simulink model "PMSM_comparison_with_matlab"  (R2023a)
settings: Solver=VariableStepAuto  StartTime=0.0  StopTime=10  MaxStep=1.0E-5  RelTol=1e-3  EnableMultiTasking=on
values from neighbouring files (symbols this model uses):
  F = 7.59e-5    (= 7.59e-05)    [initialize_motor.m]
  flux = 0.1    [initialize_motor.m]
  J = 0.00012    [initialize_motor.m]
  Ld = 0.004    [initialize_motor.m]
  Lq = 0.0035    [initialize_motor.m]
  P = 6    [initialize_motor.m]
  Rs = 2.2    [initialize_motor.m]
undefined symbols (not defined in the file or in its folder): induction_motor, sin_cos_calculator
libraries: spsACVoltageSourceLib x3, spsPermanentMagnetSynchronousMachineLib x1, spsGroundLib x1, spsThreePhaseSeriesRLCLoadLib x1, sps_lib x1
Description:
  | This model implements the model of permanent magnet synchronous motor
  | and compare it with the matlab model for verification of correctness.
  | 
  | Created by:
  | 
  | Syed Abdul Rahman Kashif
  | UET, Lahore
settings Model: Creator=kashif  LastModifiedBy=Derrick Baalaboore
settings SolverCC: AlgebraicLoopSolver=TrustRegion
settings DataIOCC: LimitDataPoints=on  SaveFormat=Array  SignalLoggingSaveFormat=ModelDataLogs  ReturnWorkspaceOutputs=off
settings OptimizationCC: ExpressionDepthLimit=2147483647  InitFltsAndDblsToZero=on  LifeSpan=inf
settings DebuggingCC: SaveWithParameterizedLinksMsg=none  UnderspecifiedInitializationDetection=Classic  MergeDetectMultiDrivingBlocksExec=none  SolverPrmCheckMsg=warning  MultiTaskCondExecSysMsg=none  FcnCallInpInsideContextMsg=warning  UnconnectedInputMsg=warning  UnconnectedOutputMsg=warning  UnconnectedLineMsg=warning  StateNameClashWarn=warning  SFUnexpectedBacktrackingDiag=warning  SFNoUnconditionalDefaultTransitionDiag=warning  SFExecutionAtInitializationDiag=none  ArithmeticOperatorsInVariantConditions=warning
settings HardwareCC: ProdBitPerPointer=32  ProdBitPerSizeT=32  ProdBitPerPtrDiffT=32  ProdLargestAtomicFloat=None  ProdIntDivRoundTo=Undefined  ProdEndianess=Unspecified  ProdWordSize=32  ProdHWDeviceType=32-bit Generic
settings ModelReferenceCC: PropagateSignalLabelsOutOfModel=off
settings SFSimCC: SimUseLocalCustomCode=off  CustomCodeUndefinedFunction=UseInterfaceOnly
settings RTWCC: RTWUseLocalCustomCode=off
settings CodeAppCC: StateflowObjectComments=on
settings GRTTargetCC: TargetLangStandard=C89/C90 (ANSI)  CombineOutputUpdateFcns=off  GRTInterface=on
settings ConfigComp: CovMetricSettings=dw  CovSaveCumulativeToWorkspaceVar=on  CovSaveSingleToWorkspaceVar=on  CovExternalEMLEnable=off

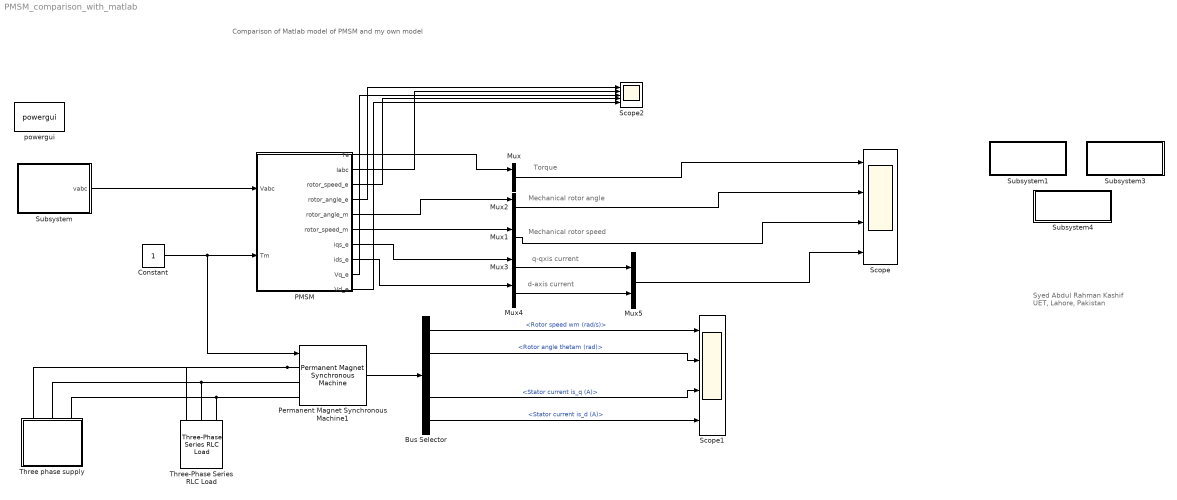
== system PMSM_comparison_with_matlab ==
  note: Torque
  note: Mechanical rotor angle
  note: Mechanical rotor speed
  note: q-qxis current
  note: d-axis current
  note: Comparison of Matlab model of PMSM and my own model
  note: Syed Abdul Rahman Kashif
      | UET, Lahore, Pakistan
  Bus Selector : BusSelector  OutputSignals=Rotor speed wm (rad/s),Rotor angle thetam (rad),Electromagnetic torque Te (N*m),Stator current is_q (A),Stator current is_d (A)
  Constant : Constant
  Mux{,1..5} (6 alike) : Mux  Inputs=2
  PMSM : Subsystem
  Permanent Magnet Synchronous Machine1 : spsPermanentMagnetSynchronousMachineLib/Permanent Magnet Synchronous Machine  NbPhases=3  FluxDistribution=Sinusoidal  RotorType=Salient-pole  MechanicalLoad=Torque Tm  PresetModel=No  ShowDetailedParameters=on  MeasurementBus=off  Resistance=1.6  Inductance=8.5e-3  dqInductances=[0.006365 0.006365]  La=0.000395  MachineConstant=Flux linkage established by magnets (V.s)  Flux=0.1852  VoltageCst=134.3663  TorqueCst=1.1112  Flat=120  Mechanical=[0.0001854 5.39e-5 4]  PolePairs=4  InitialConditions=[0,0, 0,0]  InitialConditions5ph=[0 0 0 0 0 0]  RefAngle=90 degrees behind phase A axis (modified Park)  IterativeDiscreteModel=Trapezoidal non iterative  TsBlock=-1  TsPowergui=0
  Scope : Scope  NumInputPorts=4
  Scope1 : Scope  NumInputPorts=4
  Scope2 : Scope  NumInputPorts=5
  Subsystem : Subsystem  mask{Vrms=220, f=50}
      mask prompts: f "frequency"
      mask Display: fprintf('Three phase \n Supply Vrms')
  Subsystem1 : Subsystem
      settings: OpenFcn=initialize_motor
      mask Display: fprintf('Initializing \n Data');
  Subsystem3 : Subsystem
      settings: OpenFcn=open('initialize_motor.m')
      mask Display: fprintf('Edit Data')
  Subsystem4 : Subsystem
      settings: OpenFcn=|
      | clear;
      | clc;
      | fprintf('All the Data has been cleared\n');
      mask Display: fprintf('Clear Data')
  Three phase supply : Subsystem  mask{Vrms=220, f=50}
      mask prompts: f "Frequency"
      mask Display: fprintf('Three phase \n Supply Vrms')
  Three-Phase Series RLC Load : spsThreePhaseSeriesRLCLoadLib/Three-Phase Series RLC Load  LConnTagsString=A|B|C  Configuration=Y (grounded)  NominalVoltage=220  Vabc=[1e3 1e3 1e3]  Vabcp=[1e3 1e3 1e3]  NominalFrequency=50  UnbalancedPower=off  ActivePower=100  InductivePower=0  CapacitivePower=0  Pabc=[10e3 9e3 11e3]  QLabc=[100 90 110]  QCabc=[100 90 110]  Pabcp=[10e3 9e3 11e3]  QLabcp=[100 90 110]  QCabcp=[100 90 110]  Measurements=None  LoadType=constant Z
  powergui : sps_lib/powergui  Priority=1  SimulationMode=Continuous  SampleTime=50e-6  frequency=60  Iterations=50  frequencyindice=50  Pbase=100e6  ErrMax=1e-4  UnitsV=kV  UnitsW=MW  buscounter=0  FunctionMessages=off  echomessages=off  EnableUseOfTLC=off  CurrentSourceSwitches=on  DisableSnubberDevices=off  DisableRonSwitches=off  DisableVfSwitches=off  DisplayEquations=off  AutomaticDiscreteSolvers=off  SolverType=Tustin/Backward Euler (TBE)  Interpol=off  ExternalGateDelay=off  methode=off  Ts=0  x0status=blocks  SPID=off  SwTol=0  HookPort=off  NonlinearTolerance=1e-4  nMaxIteration=100  ContinueOnMaxIteration=off  RestoreLinks=warning  ResistiveCurrentMeasurement=off  Frange=[0:2:500]  Ylog=off  Xlog=on  ShowGrid=off  save=off  variable=ZData  structure=0  ZoomFFT=on  StartTime=0.0  cycles=1  DisplayStyle=1  fundamental=60  FreqAxis=off  MaxFrequency=1000  frequencyindicesteady=1  RmsSteady=1  display=off
  wires:
  Subsystem/1(vabc) -> PMSM/1(Vabc)
  Permanent Magnet Synchronous Machine1/1 -> Bus Selector/1
  Mux/1 -> Scope/1
  Bus Selector/1 -> Scope1/1  "<Rotor speed wm (rad/s)>"
  Bus Selector/2 -> Scope1/2  "<Rotor angle thetam (rad)>"
  PMSM/1(Te) -> Mux/1
  Bus Selector/4 -> Scope1/3  "<Stator current is_q (A)>"
  Bus Selector/5 -> Scope1/4  "<Stator current is_d (A)>"
  PMSM/6(rotor_speed_m) -> Mux1/1
  PMSM/7(iqs_e) -> Mux3/1
  PMSM/5(rotor_angle_m) -> Mux2/1
  Mux2/1 -> Scope/2
  Mux1/1 -> Scope/3
  PMSM/8(ids_e) -> Mux4/1
  Mux3/1 -> Mux5/1
  Mux4/1 -> Mux5/2
  Mux5/1 -> Scope/4
  PMSM/2(Iabc) -> Scope2/2
  PMSM/3(rotor_speed_e) -> Scope2/4
  PMSM/4(rotor_angle_e) -> Scope2/1
  PMSM/9(Vq_e) -> Scope2/3
  PMSM/10(Vd_e) -> Scope2/5
  Constant/1 -> Permanent Magnet Synchronous Machine1/1, PMSM/2(Tm)
  connections:
  Permanent Magnet Synchronous Machine1/LConn1 -- Three phase supply/RConn1 -- Three-Phase Series RLC Load/LConn1
  Three phase supply/RConn2 -- Permanent Magnet Synchronous Machine1/LConn2 -- Three-Phase Series RLC Load/LConn2
  Three phase supply/RConn3 -- Permanent Magnet Synchronous Machine1/LConn3 -- Three-Phase Series RLC Load/LConn3

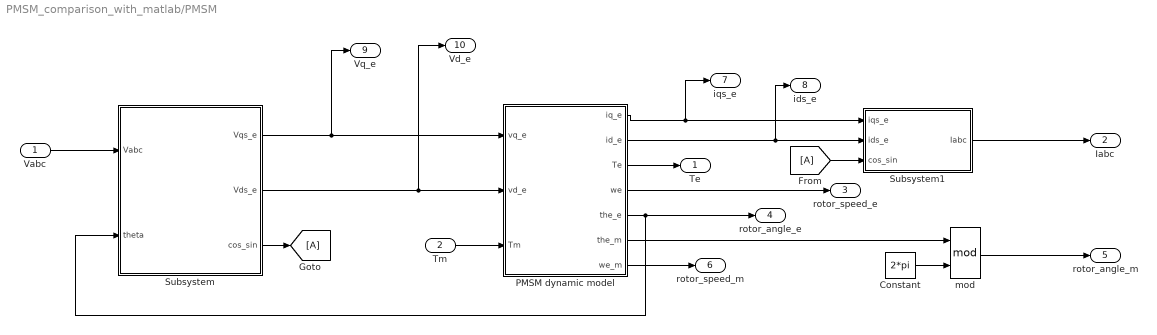
== system PMSM_comparison_with_matlab/PMSM ==
  Vabc : Inport
  Tm : Inport  Port=2
  Constant : Constant  Value=2*pi
  From : From
  Goto : Goto
  PMSM dynamic model : Subsystem
  Subsystem : Subsystem
  Subsystem1 : Subsystem
  mod : Math  Operator=mod  SignedPower=on
  Te : Outport
  Iabc : Outport  Port=2
  rotor_speed_e : Outport  Port=3
  rotor_angle_e : Outport  Port=4
  rotor_angle_m : Outport  Port=5
  rotor_speed_m : Outport  Port=6
  iqs_e : Outport  Port=7
  ids_e : Outport  Port=8
  Vq_e : Outport  Port=9
  Vd_e : Outport  Port=10
  wires:
  PMSM dynamic model/1(iq_e) -> iqs_e/1, Subsystem1/1(iqs_e)
  PMSM dynamic model/2(id_e) -> Subsystem1/2(ids_e), ids_e/1
  PMSM dynamic model/5(the_e) -> rotor_angle_e/1, Subsystem/2(theta)
  Subsystem/1(Vqs_e) -> Vq_e/1, PMSM dynamic model/1(vq_e)
  Subsystem/2(Vds_e) -> Vd_e/1, PMSM dynamic model/2(vd_e)
  PMSM dynamic model/4(we) -> rotor_speed_e/1
  PMSM dynamic model/3(Te) -> Te/1
  Vabc/1 -> Subsystem/1(Vabc)
  Tm/1 -> PMSM dynamic model/3(Tm)
  Subsystem1/1(Iabc) -> Iabc/1
  PMSM dynamic model/7(we_m) -> rotor_speed_m/1
  PMSM dynamic model/6(the_m) -> mod/1
  Constant/1 -> mod/2
  mod/1 -> rotor_angle_m/1
  Subsystem/3(cos_sin) -> Goto/1
  From/1 -> Subsystem1/3(cos_sin)

== system PMSM_comparison_with_matlab/Subsystem ==
  Mux : Mux  Inputs=3
  phase a : Sin  Amplitude=Vrms*sqrt(2)  Frequency=f*2*pi  SampleTime=0
  phase b : Sin  Amplitude=Vrms*sqrt(2)  Frequency=f*2*pi  Phase=240*pi/180  SampleTime=0
  phase c : Sin  Amplitude=Vrms*sqrt(2)  Frequency=f*2*pi  Phase=120*pi/180  SampleTime=0
  vabc : Outport
  wires:
  phase a/1 -> Mux/1
  phase b/1 -> Mux/2
  phase c/1 -> Mux/3
  Mux/1 -> vabc/1

== system PMSM_comparison_with_matlab/Subsystem1 ==

== system PMSM_comparison_with_matlab/Subsystem3 ==

== system PMSM_comparison_with_matlab/Subsystem4 ==

== system PMSM_comparison_with_matlab/Three phase supply ==
  Ground : spsGroundLib/Ground  LConnTagsString=a
  Va : spsACVoltageSourceLib/AC Voltage Source  Amplitude=Vrms*sqrt(2)  Phase=0  Frequency=f  SampleTime=0  Measurements=None  BusType=swing  Pref=10e3  Qref=0  Qmin=-inf  Qmax=+inf
  Vb : spsACVoltageSourceLib/AC Voltage Source  Amplitude=Vrms*sqrt(2)  Phase=240  Frequency=f  SampleTime=0  Measurements=None  BusType=swing  Pref=10e3  Qref=0  Qmin=-inf  Qmax=+inf
  Vc : spsACVoltageSourceLib/AC Voltage Source  Amplitude=Vrms*sqrt(2)  Phase=120  Frequency=f  SampleTime=0  Measurements=None  BusType=swing  Pref=10e3  Qref=0  Qmin=-inf  Qmax=+inf
  a : PMIOPort  Side=Right
  b : PMIOPort  Port=2  Side=Right
  c : PMIOPort  Port=3  Side=Right
  connections:
  Vb/LConn1 -- Va/LConn1 -- Ground/LConn1 -- Vc/LConn1
  a/RConn1 -- Va/RConn1
  b/RConn1 -- Vb/RConn1
  c/RConn1 -- Vc/RConn1

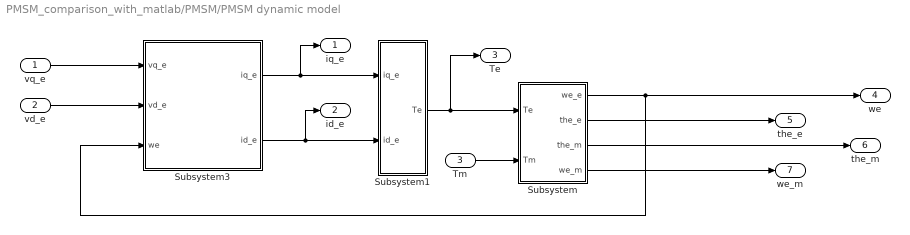
== system PMSM_comparison_with_matlab/PMSM/PMSM dynamic model ==
  vq_e : Inport
  vd_e : Inport  Port=2
  Tm : Inport  Port=3
  Subsystem : Subsystem
  Subsystem1 : Subsystem
  Subsystem3 : Subsystem
  iq_e : Outport
  id_e : Outport  Port=2
  Te : Outport  Port=3
  we : Outport  Port=4
  the_e : Outport  Port=5
  the_m : Outport  Port=6
  we_m : Outport  Port=7
  wires:
  Subsystem1/1(Te) -> Subsystem/1(Te), Te/1
  Subsystem3/1(iq_e) -> Subsystem1/1(iq_e), iq_e/1
  Subsystem3/2(id_e) -> Subsystem1/2(id_e), id_e/1
  Tm/1 -> Subsystem/2(Tm)
  vq_e/1 -> Subsystem3/1(vq_e)
  vd_e/1 -> Subsystem3/2(vd_e)
  Subsystem/2(the_e) -> the_e/1
  Subsystem/1(we_e) -> we/1, Subsystem3/3(we)
  Subsystem/3(the_m) -> the_m/1
  Subsystem/4(we_m) -> we_m/1

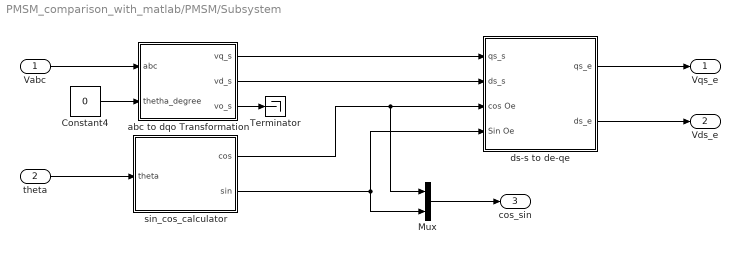
== system PMSM_comparison_with_matlab/PMSM/Subsystem ==
  Vabc : Inport
  theta : Inport  Port=2
  Constant4 : Constant  Value=0
  Mux : Mux  Inputs=2
  Terminator : Terminator
  abc to dqo Transformation : Subsystem  AncestorBlock=induction_motor/abc to dqo Transformation
      settings: LibrarySourceBlock=induction_motor/abc to dqo Transformation
  ds-s to de-qe : Subsystem  AncestorBlock=induction_motor/ds-s to de-qe
      settings: LibrarySourceBlock=induction_motor/ds-s to de-qe
  sin_cos_calculator : Subsystem  AncestorBlock=induction_motor/sin_cos_calculator
      settings: LibrarySourceBlock=induction_motor/sin_cos_calculator
  Vqs_e : Outport
  Vds_e : Outport  Port=2
  cos_sin : Outport  Port=3
  wires:
  abc to dqo Transformation/1(vq_s) -> ds-s to de-qe/1(qs_s)
  abc to dqo Transformation/2(vd_s) -> ds-s to de-qe/2(ds_s)
  Vabc/1 -> abc to dqo Transformation/1(abc)
  Constant4/1 -> abc to dqo Transformation/2(thetha_degree)
  ds-s to de-qe/1(qs_e) -> Vqs_e/1
  abc to dqo Transformation/3(vo_s) -> Terminator/1
  ds-s to de-qe/2(ds_e) -> Vds_e/1
  theta/1 -> sin_cos_calculator/1(theta)
  sin_cos_calculator/1(cos) -> ds-s to de-qe/3(cos Oe), Mux/1
  sin_cos_calculator/2(sin) -> ds-s to de-qe/4(Sin Oe), Mux/2
  Mux/1 -> cos_sin/1

== system PMSM_comparison_with_matlab/PMSM/Subsystem1 ==
  iqs_e : Inport
  ids_e : Inport  Port=2
  cos_sin : Inport  Port=3
  Constant2 : Constant  Value=0
  Demux : Demux  Outputs=2
  Subsystem : Subsystem
  de-qe to ds-qs : Subsystem  AncestorBlock=induction_motor/de-qe to ds-qs
      settings: LibrarySourceBlock=induction_motor/de-qe to ds-qs
  Iabc : Outport
  wires:
  de-qe to ds-qs/1(qs_s) -> Subsystem/1(q_s)
  de-qe to ds-qs/2(ds_s) -> Subsystem/2(d_s)
  Constant2/1 -> Subsystem/4(thetha_degree)
  Subsystem/1(abc) -> Iabc/1
  iqs_e/1 -> de-qe to ds-qs/1(qs_e)
  ids_e/1 -> de-qe to ds-qs/2(ds_e)
  Demux/1 -> de-qe to ds-qs/3(cos Oe)
  ? -> Subsystem/3(o_s)
  Demux/2 -> de-qe to ds-qs/4(Sin Oe)
  cos_sin/1 -> Demux/1

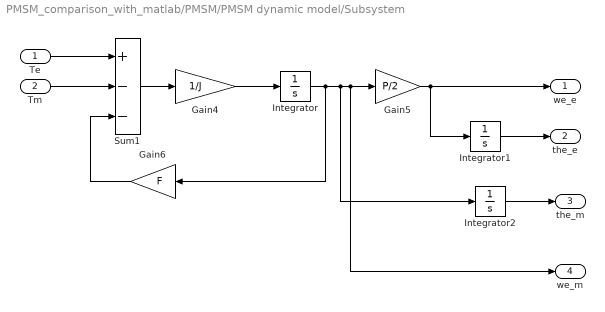
== system PMSM_comparison_with_matlab/PMSM/PMSM dynamic model/Subsystem ==
  Te : Inport
  Tm : Inport  Port=2
  Gain4 : Gain  Gain=1/J  SaturateOnIntegerOverflow=on  OutDataTypeStr=Inherit: Same as input  ParamDataTypeStr=Inherit: Same as input
  Gain5 : Gain  Gain=P/2  SaturateOnIntegerOverflow=on  OutDataTypeStr=Inherit: Same as input  ParamDataTypeStr=Inherit: Same as input
  Gain6 : Gain  Gain=F  SaturateOnIntegerOverflow=on  OutDataTypeStr=Inherit: Same as input  ParamDataTypeStr=Inherit: Same as input
  Integrator : Integrator
  Integrator1 : Integrator
  Integrator2 : Integrator
  Sum1 : Sum  Inputs=+--  InputSameDT=on  SaturateOnIntegerOverflow=on  OutDataTypeStr=Inherit: Same as first input
  we_e : Outport
  the_e : Outport  Port=2
  the_m : Outport  Port=3
  we_m : Outport  Port=4
  wires:
  Te/1 -> Sum1/1
  Tm/1 -> Sum1/2
  Sum1/1 -> Gain4/1
  Gain4/1 -> Integrator/1
  Integrator/1 -> Gain6/1, Integrator2/1, Gain5/1, we_m/1
  Gain6/1 -> Sum1/3
  Gain5/1 -> Integrator1/1, we_e/1
  Integrator1/1 -> the_e/1
  Integrator2/1 -> the_m/1

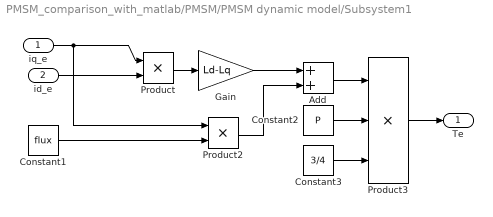
== system PMSM_comparison_with_matlab/PMSM/PMSM dynamic model/Subsystem1 ==
  iq_e : Inport
  id_e : Inport  Port=2
  Add : Sum
  Constant1 : Constant  Value=flux
  Constant2 : Constant  Value=P
  Constant3 : Constant  Value=3/4
  Gain : Gain  Gain=Ld-Lq
  Product : Product  RndMeth=Zero
  Product2 : Product  RndMeth=Zero
  Product3 : Product  Inputs=3  RndMeth=Zero
  Te : Outport
  wires:
  iq_e/1 -> Product/1, Product2/1
  id_e/1 -> Product/2
  Product/1 -> Gain/1
  Constant1/1 -> Product2/2
  Gain/1 -> Add/1
  Product2/1 -> Add/2
  Add/1 -> Product3/1
  Constant2/1 -> Product3/2
  Constant3/1 -> Product3/3
  Product3/1 -> Te/1

== system PMSM_comparison_with_matlab/PMSM/PMSM dynamic model/Subsystem3 ==
  vq_e : Inport
  vd_e : Inport  Port=2
  we : Inport  Port=3
  Subsystem1 : Subsystem
  Subsystem2 : Subsystem
  iq_e : Outport
  id_e : Outport  Port=2
  wires:
  vq_e/1 -> Subsystem1/3(vq)
  vd_e/1 -> Subsystem2/3(vd)
  we/1 -> Subsystem1/2(we), Subsystem2/2(we)
  Subsystem1/1(iq) -> Subsystem2/1(iq), iq_e/1
  Subsystem2/1(id) -> Subsystem1/1(id), id_e/1

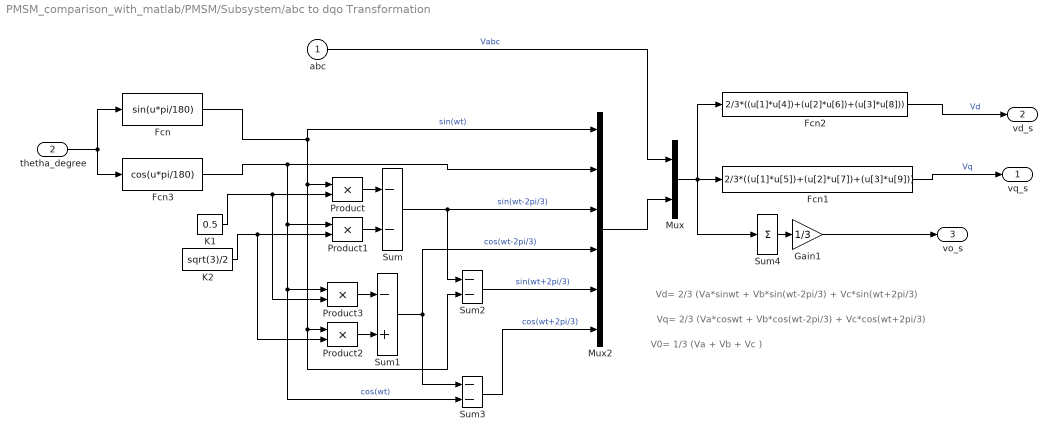
== system PMSM_comparison_with_matlab/PMSM/Subsystem/abc to dqo Transformation ==
  note: Vq= 2/3 (Va*coswt + Vb*cos(wt-2pi/3) + Vc*cos(wt+2pi/3)
  note: Vd= 2/3 (Va*sinwt + Vb*sin(wt-2pi/3) + Vc*sin(wt+2pi/3)
  note: V0= 1/3 (Va + Vb + Vc )
  abc : Inport  PortDimensions=3
  thetha_degree : Inport  Port=2
  Fcn : Fcn  Expr=sin(u*pi/180)
  Fcn1 : Fcn  Expr=2/3*((u[1]*u[5])+(u[2]*u[7])+(u[3]*u[9]))
  Fcn2 : Fcn  Expr=2/3*((u[1]*u[4])+(u[2]*u[6])+(u[3]*u[8]))
  Fcn3 : Fcn  Expr=cos(u*pi/180)
  Gain1 : Gain  Gain=1/3  SaturateOnIntegerOverflow=on  OutDataTypeStr=Inherit: Same as input  ParamDataTypeStr=Inherit: Same as input
  K1 : Constant  Value=0.5
  K2 : Constant  Value=sqrt(3)/2
  Mux : Mux  Inputs=2
  Mux2 : Mux  Inputs=6
  Product{,1..3} (4 alike) : Product  InputSameDT=on  SaturateOnIntegerOverflow=on  OutDataTypeStr=Inherit: Same as first input
  Sum : Sum  Inputs=--  InputSameDT=on  SaturateOnIntegerOverflow=on  OutDataTypeStr=Inherit: Same as first input
  Sum1 : Sum  Inputs=-+  InputSameDT=on  SaturateOnIntegerOverflow=on  OutDataTypeStr=Inherit: Same as first input
  Sum2 : Sum  Inputs=--  InputSameDT=on  SaturateOnIntegerOverflow=on  OutDataTypeStr=Inherit: Same as first input
  Sum3 : Sum  Inputs=--  InputSameDT=on  SaturateOnIntegerOverflow=on  OutDataTypeStr=Inherit: Same as first input
  Sum4 : Sum  Inputs=1  InputSameDT=on  SaturateOnIntegerOverflow=on  OutDataTypeStr=Inherit: Same as first input
  vq_s : Outport
  vd_s : Outport  Port=2
  vo_s : Outport  Port=3
  wires:
  Fcn2/1 -> vd_s/1  "Vd"
  Fcn1/1 -> vq_s/1  "Vq"
  abc/1 -> Mux/1  "Vabc"
  Mux2/1 -> Mux/2
  Fcn3/1 -> Sum3/2, Product3/1, Product1/1, Mux2/2  "cos(wt)"
  Fcn/1 -> Product/1, Product2/1, Sum2/2, Mux2/1  "sin(wt)"
  Product/1 -> Sum/1
  Product1/1 -> Sum/2
  Product3/1 -> Sum1/1
  Product2/1 -> Sum1/2
  Sum3/1 -> Mux2/6  "cos(wt+2pi/3)"
  Sum2/1 -> Mux2/5  "sin(wt+2pi/3)"
  K1/1 -> Product/2, Product3/2
  K2/1 -> Product1/2, Product2/2
  Sum/1 -> Mux2/3, Sum2/1  "sin(wt-2pi/3)"
  Sum1/1 -> Mux2/4, Sum3/1  "cos(wt-2pi/3)"
  Mux/1 -> Fcn2/1, Fcn1/1, Sum4/1
  Sum4/1 -> Gain1/1
  Gain1/1 -> vo_s/1
  thetha_degree/1 -> Fcn3/1, Fcn/1

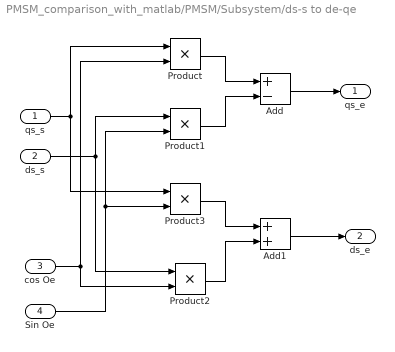
== system PMSM_comparison_with_matlab/PMSM/Subsystem/ds-s to de-qe ==
  qs_s : Inport
  ds_s : Inport  Port=2
  cos Oe : Inport  Port=3
  Sin Oe : Inport  Port=4
  Add : Sum  Inputs=+-
  Add1 : Sum
  Product{,1..3} (4 alike) : Product  RndMeth=Zero
  qs_e : Outport
  ds_e : Outport  Port=2
  wires:
  Product/1 -> Add/1
  Product1/1 -> Add/2
  Product2/1 -> Add1/2
  Product3/1 -> Add1/1
  Add1/1 -> ds_e/1
  Add/1 -> qs_e/1
  Sin Oe/1 -> Product1/2, Product3/2
  ds_s/1 -> Product1/1, Product2/1
  cos Oe/1 -> Product/2, Product2/2
  qs_s/1 -> Product/1, Product3/1

== system PMSM_comparison_with_matlab/PMSM/Subsystem/sin_cos_calculator ==
  theta : Inport
  Fcn : Fcn  Expr=sin(u)
  Fcn1 : Fcn  Expr=cos(u)
  cos : Outport
  sin : Outport  Port=2
  wires:
  Fcn1/1 -> cos/1
  Fcn/1 -> sin/1
  theta/1 -> Fcn/1, Fcn1/1

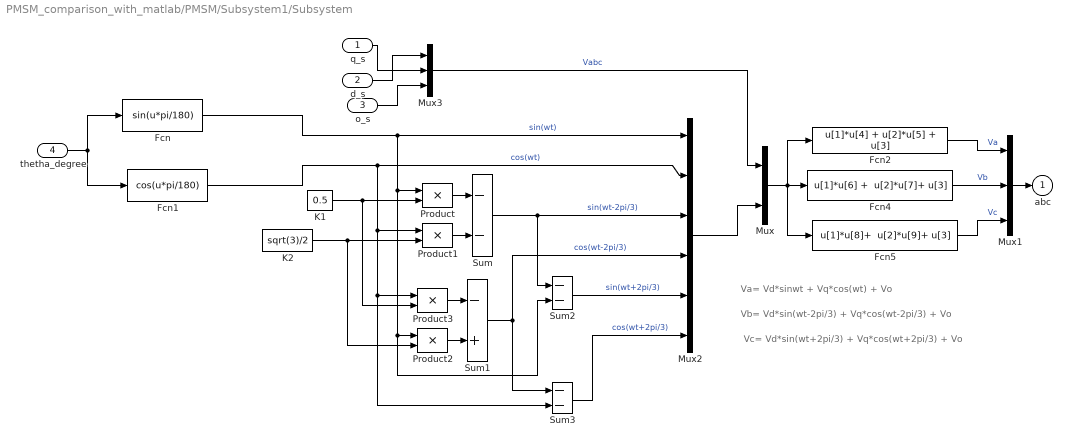
== system PMSM_comparison_with_matlab/PMSM/Subsystem1/Subsystem ==
  note: Va= Vd*sinwt + Vq*cos(wt) + Vo
  note: Vb= Vd*sin(wt-2pi/3) + Vq*cos(wt-2pi/3) + Vo
  note: Vc= Vd*sin(wt+2pi/3) + Vq*cos(wt+2pi/3) + Vo
  q_s : Inport
  d_s : Inport  Port=2
  o_s : Inport  Port=3
  thetha_degree : Inport  Port=4
  Fcn : Fcn  Expr=sin(u*pi/180)
  Fcn1 : Fcn  Expr=cos(u*pi/180)
  Fcn2 : Fcn  Expr="u[1]*u[4] +  u[2]*u[5] + u[3]"
  Fcn4 : Fcn  Expr="u[1]*u[6] +  u[2]*u[7]+ u[3]"
  Fcn5 : Fcn  Expr="u[1]*u[8]+  u[2]*u[9]+ u[3]"
  K1 : Constant  Value=0.5
  K2 : Constant  Value=sqrt(3)/2
  Mux : Mux  Inputs=2
  Mux1 : Mux  Inputs=3
  Mux2 : Mux  Inputs=6
  Mux3 : Mux  Inputs=3
  Product{,1..3} (4 alike) : Product  InputSameDT=on  SaturateOnIntegerOverflow=on  OutDataTypeStr=Inherit: Same as first input
  Sum : Sum  Inputs=--  InputSameDT=on  SaturateOnIntegerOverflow=on  OutDataTypeStr=Inherit: Same as first input
  Sum1 : Sum  Inputs=-+  InputSameDT=on  SaturateOnIntegerOverflow=on  OutDataTypeStr=Inherit: Same as first input
  Sum2 : Sum  Inputs=--  InputSameDT=on  SaturateOnIntegerOverflow=on  OutDataTypeStr=Inherit: Same as first input
  Sum3 : Sum  Inputs=--  InputSameDT=on  SaturateOnIntegerOverflow=on  OutDataTypeStr=Inherit: Same as first input
  abc : Outport  InitialOutput=0
  wires:
  o_s/1 -> Mux3/3
  q_s/1 -> Mux3/2
  d_s/1 -> Mux3/1
  Fcn5/1 -> Mux1/3  "Vc"
  Fcn2/1 -> Mux1/1  "Va"
  Mux1/1 -> abc/1
  Mux/1 -> Fcn4/1, Fcn2/1, Fcn5/1
  Sum1/1 -> Sum3/1, Mux2/4  "cos(wt-2pi/3)"
  Sum/1 -> Sum2/1, Mux2/3  "sin(wt-2pi/3)"
  K2/1 -> Product2/2, Product1/2
  K1/1 -> Product3/2, Product/2
  Sum2/1 -> Mux2/5  "sin(wt+2pi/3)"
  Sum3/1 -> Mux2/6  "cos(wt+2pi/3)"
  Product2/1 -> Sum1/2
  Product3/1 -> Sum1/1
  Product1/1 -> Sum/2
  Product/1 -> Sum/1
  Mux2/1 -> Mux/2
  Mux3/1 -> Mux/1  "Vabc"
  Fcn4/1 -> Mux1/2  "Vb"
  Fcn1/1 -> Mux2/2, Product1/1, Product3/1, Sum3/2  "cos(wt)"
  thetha_degree/1 -> Fcn/1, Fcn1/1
  Fcn/1 -> Mux2/1, Product/1, Sum2/2, Product2/1  "sin(wt)"

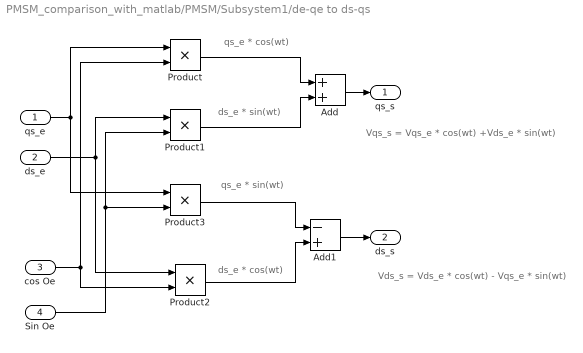
== system PMSM_comparison_with_matlab/PMSM/Subsystem1/de-qe to ds-qs ==
  note: Vds_s = Vds_e * cos(wt) - Vqs_e * sin(wt)
  note: Vqs_s = Vqs_e * cos(wt) +Vds_e * sin(wt)
  note: ds_e * cos(wt)
  note: qs_e * sin(wt)
  note: ds_e * sin(wt)
  note: qs_e * cos(wt)
  qs_e : Inport
  ds_e : Inport  Port=2
  cos Oe : Inport  Port=3
  Sin Oe : Inport  Port=4
  Add : Sum
  Add1 : Sum  Inputs=-+
  Product{,1..3} (4 alike) : Product  RndMeth=Zero
  qs_s : Outport
  ds_s : Outport  Port=2
  wires:
  Product/1 -> Add/1
  Product1/1 -> Add/2
  Product2/1 -> Add1/2
  Product3/1 -> Add1/1
  Add1/1 -> ds_s/1
  Add/1 -> qs_s/1
  Sin Oe/1 -> Product1/2, Product3/2
  ds_e/1 -> Product1/1, Product2/1
  cos Oe/1 -> Product/2, Product2/2
  qs_e/1 -> Product/1, Product3/1

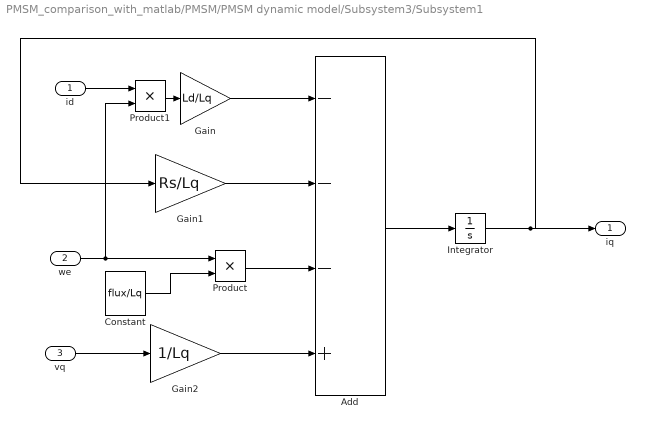
== system PMSM_comparison_with_matlab/PMSM/PMSM dynamic model/Subsystem3/Subsystem1 ==
  id : Inport
  we : Inport  Port=2
  vq : Inport  Port=3
  Add : Sum  Inputs=---+
  Constant : Constant  Value=flux/Lq
  Gain : Gain  Gain=Ld/Lq
  Gain1 : Gain  Gain=Rs/Lq
  Gain2 : Gain  Gain=1/Lq
  Integrator : Integrator
  Product : Product  RndMeth=Zero
  Product1 : Product  RndMeth=Zero
  iq : Outport
  wires:
  vq/1 -> Gain2/1
  Gain/1 -> Add/1
  Gain1/1 -> Add/2
  Gain2/1 -> Add/4
  Add/1 -> Integrator/1
  Integrator/1 -> Gain1/1, iq/1
  Product/1 -> Add/3
  we/1 -> Product/1, Product1/2
  Constant/1 -> Product/2
  Product1/1 -> Gain/1
  id/1 -> Product1/1

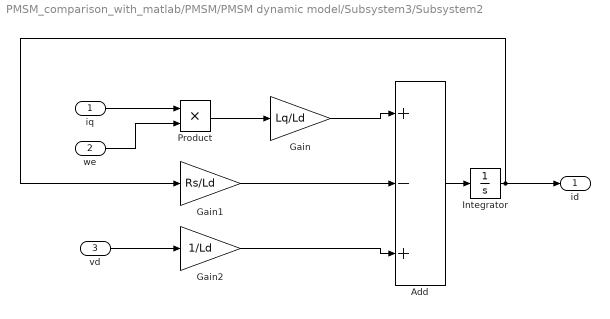
== system PMSM_comparison_with_matlab/PMSM/PMSM dynamic model/Subsystem3/Subsystem2 ==
  iq : Inport
  we : Inport  Port=2
  vd : Inport  Port=3
  Add : Sum  Inputs=+-+
  Gain : Gain  Gain=Lq/Ld
  Gain1 : Gain  Gain=Rs/Ld
  Gain2 : Gain  Gain=1/Ld
  Integrator : Integrator
  Product : Product  RndMeth=Zero
  id : Outport
  wires:
  iq/1 -> Product/1
  we/1 -> Product/2
  Product/1 -> Gain/1
  Gain/1 -> Add/1
  Add/1 -> Integrator/1
  Gain1/1 -> Add/2
  vd/1 -> Gain2/1
  Gain2/1 -> Add/3
  Integrator/1 -> Gain1/1, id/1
